simulink model "Simo"  (R2021b)
settings: Solver=ode113  StartTime=0.0  StopTime=500.0  MaxStep=20  MinStep=10  RelTol=1e-3
settings Model: PacingRate=11  Creator=user  LastModifiedBy=user

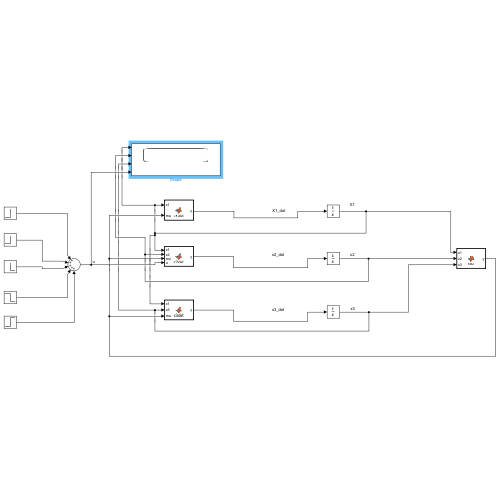
[thumbnail: Simulink's stored preview of the top-level diagram]
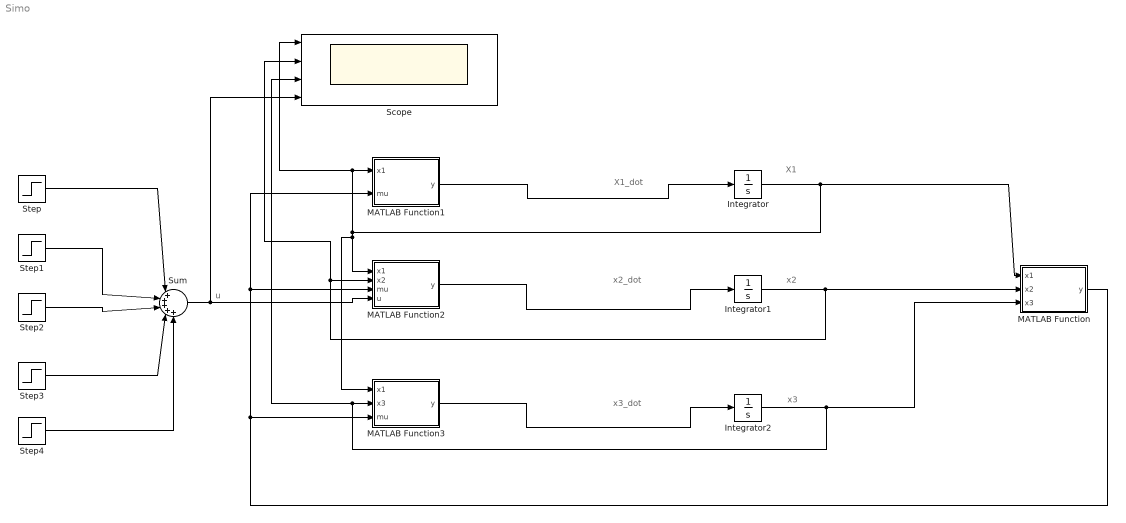
== system Simo ==
  note: u
  note: x3
  note: x2
  note: X1
  note: X1_dot
  note: x2_dot
  note: x3_dot
  Integrator : Integrator
  Integrator1 : Integrator
  Integrator2 : Integrator
  MATLAB Function : MATLAB Function  TreatAsAtomicUnit=on
  MATLAB Function1 : MATLAB Function  TreatAsAtomicUnit=on
  MATLAB Function2 : MATLAB Function  TreatAsAtomicUnit=on
  MATLAB Function3 : MATLAB Function  TreatAsAtomicUnit=on
  Scope : Scope  NumInputPorts=4
  Step : Step  Time=0  After=25  SampleTime=0
  Step1 : Step  Time=100  After=5  SampleTime=0
  Step2 : Step  Time=200  After=-5  SampleTime=0
  Step3 : Step  Time=300  After=-5  SampleTime=0
  Step4 : Step  Time=400  After=5  SampleTime=0
  Sum : Sum  Inputs=|+++++
  wires:
  MATLAB Function1/1(y) -> Integrator/1
  MATLAB Function3/1(y) -> Integrator2/1
  MATLAB Function/1(y) -> MATLAB Function3/3(mu), MATLAB Function1/2(mu), MATLAB Function2/3(mu)
  MATLAB Function2/1(y) -> Integrator1/1
  Integrator2/1 -> Scope/3, MATLAB Function3/2(x3), MATLAB Function/3(x3)
  Integrator1/1 -> Scope/2, MATLAB Function2/2(x2), MATLAB Function/2(x2)
  Sum/1 -> Scope/4, MATLAB Function2/4(u)
  Step4/1 -> Sum/5
  Step3/1 -> Sum/4
  Step2/1 -> Sum/3
  Step1/1 -> Sum/2
  Step/1 -> Sum/1
  Integrator/1 -> MATLAB Function3/1(x1), MATLAB Function2/1(x1), MATLAB Function1/1(x1), Scope/1, MATLAB Function/1(x1)

== matlab function Simo/MATLAB Function1 ==
  data: x1 input; y output; mu input
function y = x1dot(x1,mu)

y = -0.15*x1+mu*x1;

== matlab function Simo/MATLAB Function ==
  data: x1 input; y output; x2 input; x3 input
function y = mu(x1,x2,x3)

y = ( 0.48*(1-0.02*x3)*x2 )/( 1.2+x2+( (x2^2)/22 ) );

== matlab function Simo/MATLAB Function2 ==
  data: x1 input; y output; x2 input; mu input; u input
function y = x2dot(x1,x2,mu,u)

y = 0.15*(u - x2)-2.5*mu*x1;

== matlab function Simo/MATLAB Function3 ==
  data: x1 input; x3 input; mu input; y output
function y = x3dot(x1,x3,mu)

y = -0.15*x3+(2.2*mu+0.2)*x1;
